simulink model "unfulldeminsionscope"  (R2016b)
settings: Solver=VariableStepAuto  StartTime=0.0  StopTime=10.0  RelTol=1e-3
settings Model: Creator=gz199  LastModifiedBy=gz199

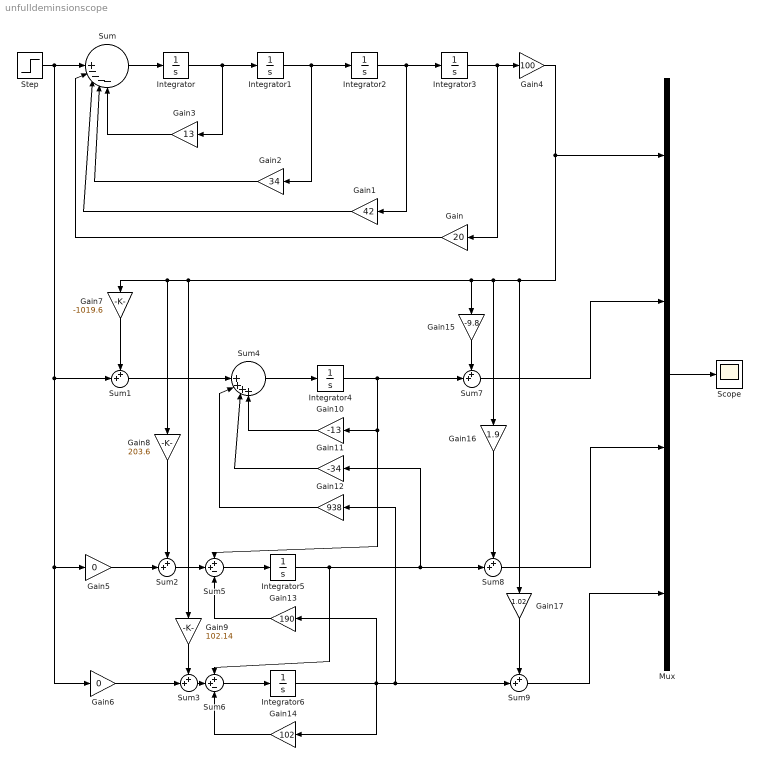
== system unfulldeminsionscope ==
  Gain : Gain  Gain=20
  Gain1 : Gain  Gain=42
  Gain10 : Gain  Gain=-13
  Gain11 : Gain  Gain=-34
  Gain12 : Gain  Gain=938
  Gain13 : Gain  Gain=190
  Gain14 : Gain  Gain=102
  Gain15 : Gain  Gain=-9.8
  Gain16 : Gain  Gain=1.9
  Gain17 : Gain  Gain=1.02
  Gain2 : Gain  Gain=34
  Gain3 : Gain  Gain=13
  Gain4 : Gain  Gain=100
  Gain5 : Gain  Gain=0
  Gain6 : Gain  Gain=0
  Gain7 : Gain  Gain=-1019.6
  Gain8 : Gain  Gain=203.6
  Gain9 : Gain  Gain=102.14
  Integrator{,1..6} (7 alike) : Integrator
  Mux : Mux
  Scope : Scope
  Step : Step  Time=0  SampleTime=0
  Sum : Sum  Inputs=||||+----
  Sum{1..3,7..9} (6 alike) : Sum  Inputs=++|
  Sum4 : Sum  Inputs=|||++++
  Sum5 : Sum  Inputs=++-
  Sum6 : Sum  Inputs=++-
  wires:
  Integrator/1 -> Gain3/1, Integrator1/1
  Integrator1/1 -> Gain2/1, Integrator2/1
  Integrator2/1 -> Gain1/1, Integrator3/1
  Sum/1 -> Integrator/1
  Gain/1 -> Sum/2
  Gain3/1 -> Sum/5
  Gain2/1 -> Sum/4
  Gain1/1 -> Sum/3
  Integrator3/1 -> Gain4/1, Gain/1
  Gain4/1 -> Mux/1, Gain16/1, Gain15/1, Gain9/1, Gain8/1, Gain7/1, Gain17/1
  Step/1 -> Gain6/1, Gain5/1, Sum1/2, Sum/1
  Gain6/1 -> Sum3/2
  Gain5/1 -> Sum2/2
  Gain7/1 -> Sum1/1
  Gain8/1 -> Sum2/1
  Gain9/1 -> Sum3/1
  Sum1/1 -> Sum4/1
  Sum4/1 -> Integrator4/1
  Sum5/1 -> Integrator5/1
  Sum6/1 -> Integrator6/1
  Integrator4/1 -> Sum7/2, Gain10/1, Sum5/1
  Gain10/1 -> Sum4/4
  Gain11/1 -> Sum4/3
  Gain12/1 -> Sum4/2
  Integrator5/1 -> Sum6/1, Sum8/2, Gain11/1
  Integrator6/1 -> Gain13/1, Gain14/1, Sum9/2, Gain12/1
  Sum2/1 -> Sum5/2
  Sum3/1 -> Sum6/2
  Gain13/1 -> Sum5/3
  Gain14/1 -> Sum6/3
  Gain15/1 -> Sum7/1
  Gain16/1 -> Sum8/1
  Gain17/1 -> Sum9/1
  Sum9/1 -> Mux/4
  Sum8/1 -> Mux/3
  Sum7/1 -> Mux/2
  Mux/1 -> Scope/1
